simulink model "RC_DOB_mdl"  (Simulink 9.1)
settings: Solver=ode3  StartTime=0.0  StopTime=NmaxTs*Ts  FixedStep=Ts  RelTol=1e-3  EnableMultiTasking=on
values from neighbouring files (symbols this model uses):
  alpha_end = 0.999    [main_RC_DOB.m]
  alpha_init = 0    [main_RC_DOB.m]
  alpha_judge = 0.01    [main_RC_DOB.m]
  alpha_middle = 0.99    [main_RC_DOB.m]
  alpha_rate1 = 0.9    [main_RC_DOB.m]
  alpha_rate2 = 0.95    [main_RC_DOB.m]
  codeQ_gain = 0    [main_RC_DOB.m]
  d_DOB = PnZPETinverse.delaySteps    [main_RC_DOB.m]
  filterQ_gain = 1    [main_RC_DOB.m]
  g_flutter = 1    [main_RC_DOB.m]
  g_nb = 1    [main_RC_DOB.m]
  g_rro = 1    [main_RC_DOB.m]
  g_sensor = 1    [main_RC_DOB.m]
  g_torque = 1    [main_RC_DOB.m]
  loopgain = 1+loopgain_pt(jj)    [main_RC_DOB.m]
  m = d_DOB    [main_RC_DOB.m]
  RRO = SetRRO(Tsim,PlantData)    [distDefine.m]
  switch_DOB = 1    [main_RC_DOB.m]
  t_NBon = NBm/120    (= 0)    [distDefine.m]
  t_Qon = (NBm+3-NBm)/120    (= 0.025)    [distDefine.m]
  Tc = Ts    [distDefine.m]
  Ts = PlantData.Ts    [distDefine.m]    (also in main_RC_DOB.m)
undefined symbols (not defined in the file or in its folder): FlutterDist, ForceDist, MNDist, n_lplp, PlantData, SensorNoise
libraries: cstblocks x6
settings Model: Creator=Max  LastModifiedBy=daw15004
settings DataIOCC: LimitDataPoints=on  SignalLoggingSaveFormat=ModelDataLogs  SignalLoggingName=sigsOut
settings OptimizationCC: ExpressionDepthLimit=2147483647  InitFltsAndDblsToZero=on
settings DebuggingCC: SaveWithParameterizedLinksMsg=none  SignalResolutionControl=TryResolveAllWithWarning  MultiTaskDSMMsg=warning  MultiTaskCondExecSysMsg=none  FcnCallInpInsideContextMsg=warning  StateNameClashWarn=warning
settings HardwareCC: TargetUnknown=on
settings SFSimCC: SimParseCustomCode=off
settings GRTTargetCC: GeneratePreprocessorConditionals=Disable all
settings ConfigComp: CovSFcnEnable=off

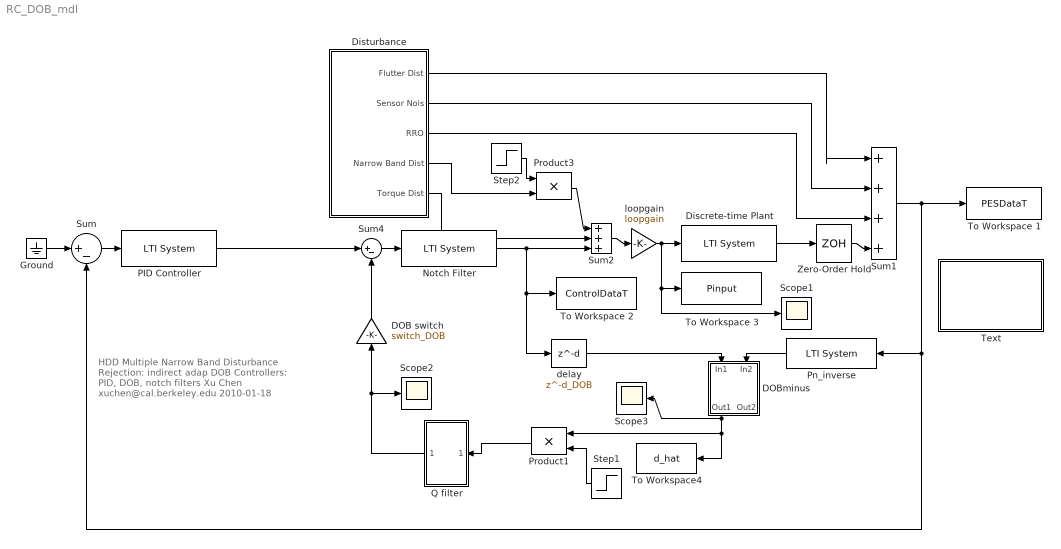
== system RC_DOB_mdl ==
  note: HDD Multiple Narrow Band
      | Disturbance Rejection: indirect adap DOB
      | Controllers: PID, DOB, notch filters
      | Xu Chen xuchen@cal.berkeley.edu
      | 2010-01-18
  DOB switch : Gain  Gain=switch_DOB  SaturateOnIntegerOverflow=on  OutDataTypeStr=Inherit: Same as input  ParamDataTypeStr=Inherit: Same as input
  DOBminus : Subsystem
  Discrete-time Plant : cstblocks/LTI System  sys=sysd_P  IC=0
  Disturbance : Subsystem
  Ground : Ground
  Notch Filter : cstblocks/LTI System  sys=sys_C2  IC=[]
  PID Controller : cstblocks/LTI System  sys=sys_C1  IC=[]
  Pn_inverse : cstblocks/LTI System  sys=G_n_inv0  IC=[]
  Product1 : Product  SaturateOnIntegerOverflow=on  OutDataTypeStr=Inherit: Same as first input
  Product3 : Product  SaturateOnIntegerOverflow=on  OutDataTypeStr=Inherit: Same as first input
  Q filter : Subsystem
  Scope1 : Scope
  Scope2 : Scope
  Scope3 : Scope
  Step1 : Step  Time=t_Qon  SampleTime=Ts
  Step2 : Step  Time=t_NBon  SampleTime=Ts
  Sum : Sum  Inputs=|+-  SaturateOnIntegerOverflow=on
  Sum1 : Sum  Inputs=+++|+  SaturateOnIntegerOverflow=on
  Sum2 : Sum  Inputs=+++  SaturateOnIntegerOverflow=on
  Sum4 : Sum  Inputs=|+-
  Text : Subsystem
      mask Display: disp('Double click here\n for help to run\nthis simulation')
  To Workspace 1 : ToWorkspace  VariableName=PESDataT  SaveFormat=Structure With Time  SampleTime=Ts
      settings: MaxDataPoints=NmaxTs
  To Workspace 2 : ToWorkspace  VariableName=ControlDataT  SaveFormat=Structure With Time  SampleTime=Tc
      settings: MaxDataPoints=NmaxTc
  To Workspace 3 : ToWorkspace  VariableName=Pinput  SaveFormat=Structure With Time  SampleTime=Tc
      settings: MaxDataPoints=NmaxTc
  To Workspace4 : ToWorkspace  VariableName=d_hat  SaveFormat=Structure With Time  SampleTime=-1
  Zero-Order Hold : ZeroOrderHold  SampleTime=Ts
  delay : Delay  DelayLength=d_DOB  InputProcessing=Inherited
  loopgain : Gain  Gain=loopgain  SaturateOnIntegerOverflow=on  OutDataTypeStr=Inherit: Same as input  ParamDataTypeStr=Inherit: Same as input
  wires:
  Ground/1 -> Sum/1
  Sum/1 -> PID Controller/1
  Sum1/1 -> To Workspace 1/1, Pn_inverse/1, Sum/2
  Disturbance/2(Sensor Nois) -> Sum1/2
  Disturbance/1(Flutter Dist) -> Sum1/1
  Disturbance/3(RRO) -> Sum1/3
  loopgain/1 -> Discrete-time Plant/1, To Workspace 3/1, Scope1/1
  Discrete-time Plant/1 -> Zero-Order Hold/1
  Zero-Order Hold/1 -> Sum1/4
  PID Controller/1 -> Sum4/1
  DOB switch/1 -> Sum4/2
  Sum2/1 -> loopgain/1
  Step2/1 -> Product3/1
  Disturbance/4(Narrow Band Dist) -> Product3/2
  Product3/1 -> Sum2/1
  Disturbance/5(Torque Dist) -> Sum2/2
  Sum4/1 -> Notch Filter/1
  Step1/1 -> Product1/2
  Product1/1 -> Q filter/1(In1)
  Q filter/1(Out1) -> DOB switch/1, Scope2/1
  delay/1 -> DOBminus/1(In1)
  Pn_inverse/1 -> DOBminus/2(In2)
  DOBminus/1(Out1) -> Scope3/1, Product1/1, To Workspace4/1
  Notch Filter/1 -> Sum2/3, To Workspace 2/1, delay/1

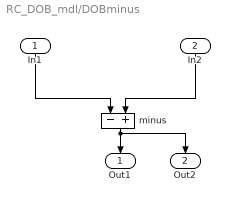
== system RC_DOB_mdl/DOBminus ==
  In1 : Inport
  In2 : Inport  Port=2
  minus : Sum  Inputs=-+
  Out1 : Outport
  Out2 : Outport  Port=2
  wires:
  In1/1 -> minus/1
  In2/1 -> minus/2
  minus/1 -> Out1/1, Out2/1

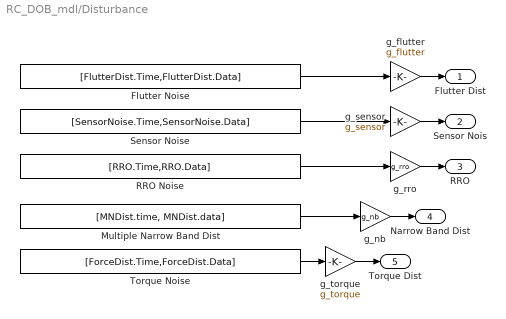
== system RC_DOB_mdl/Disturbance ==
  Flutter Noise : FromWorkspace  VariableName=[FlutterDist.Time,FlutterDist.Data]  SampleTime=FlutterDist.Ts  Interpolate=off  OutputAfterFinalValue=Setting to zero
  Multiple Narrow Band Dist : FromWorkspace  VariableName=[MNDist.time, MNDist.data]  SampleTime=MNDist.Ts  Interpolate=off  OutputAfterFinalValue=Setting to zero
  RRO Noise : FromWorkspace  VariableName=[RRO.Time,RRO.Data]  SampleTime=RRO.Ts  Interpolate=off  OutputAfterFinalValue=Setting to zero
  Sensor Noise : FromWorkspace  VariableName=[SensorNoise.Time,SensorNoise.Data]  SampleTime=SensorNoise.Ts  Interpolate=off  OutputAfterFinalValue=Setting to zero
  Torque Noise : FromWorkspace  VariableName=[ForceDist.Time,ForceDist.Data]  SampleTime=ForceDist.Ts  Interpolate=off  OutputAfterFinalValue=Setting to zero
  g_flutter : Gain  Gain=g_flutter  SaturateOnIntegerOverflow=on  OutDataTypeStr=Inherit: Same as input  ParamDataTypeStr=Inherit: Same as input
  g_nb : Gain  Gain=g_nb  SaturateOnIntegerOverflow=on  OutDataTypeStr=Inherit: Same as input  ParamDataTypeStr=Inherit: Same as input
  g_rro : Gain  Gain=g_rro  SaturateOnIntegerOverflow=on  OutDataTypeStr=Inherit: Same as input  ParamDataTypeStr=Inherit: Same as input
  g_sensor : Gain  Gain=g_sensor  SaturateOnIntegerOverflow=on  OutDataTypeStr=Inherit: Same as input  ParamDataTypeStr=Inherit: Same as input
  g_torque : Gain  Gain=g_torque  SaturateOnIntegerOverflow=on  OutDataTypeStr=Inherit: Same as input  ParamDataTypeStr=Inherit: Same as input
  Flutter Dist : Outport
  Sensor Nois : Outport  Port=2
  RRO : Outport  Port=3
  Narrow Band Dist : Outport  Port=4
  Torque Dist : Outport  Port=5
  wires:
  Multiple Narrow Band Dist/1 -> g_nb/1
  RRO Noise/1 -> g_rro/1
  Flutter Noise/1 -> g_flutter/1
  Sensor Noise/1 -> g_sensor/1
  Torque Noise/1 -> g_torque/1
  g_flutter/1 -> Flutter Dist/1
  g_sensor/1 -> Sensor Nois/1
  g_rro/1 -> RRO/1
  g_nb/1 -> Narrow Band Dist/1
  g_torque/1 -> Torque Dist/1

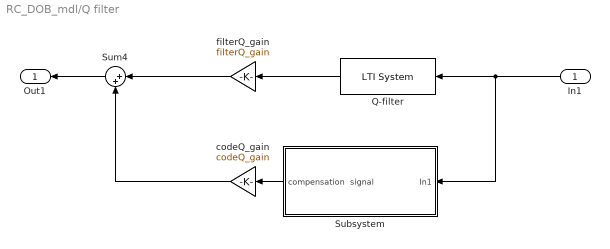
== system RC_DOB_mdl/Q filter ==
  In1 : Inport
  Q-filter : cstblocks/LTI System  sys=Q  IC=[]
  Subsystem : Subsystem
  Sum4 : Sum  Inputs=|++
  codeQ_gain : Gain  Gain=codeQ_gain  SaturateOnIntegerOverflow=on  OutDataTypeStr=Inherit: Same as input  ParamDataTypeStr=Inherit: Same as input
  filterQ_gain : Gain  Gain=filterQ_gain  SaturateOnIntegerOverflow=on  OutDataTypeStr=Inherit: Same as input  ParamDataTypeStr=Inherit: Same as input
  Out1 : Outport
  wires:
  In1/1 -> Q-filter/1, Subsystem/1(In1)
  Q-filter/1 -> filterQ_gain/1
  Subsystem/1(compensation  signal) -> codeQ_gain/1
  filterQ_gain/1 -> Sum4/1
  Sum4/1 -> Out1/1
  codeQ_gain/1 -> Sum4/2

== system RC_DOB_mdl/Text ==
  note: 3). The initial estimates (the initial conditions for the
      | integrator in the estimation algorithm block)
  note: 2). The adaptive gains (the parameters Gain and Gain1
      | in the estimation algorithm block)
  note: You can change the following parameters before
      | running the simulation and see their effects on the
      | estimator performance:
  note: This simulink program is used to implement the adaptive parallel
      | estimator in Multiple narrow band disturbance rejection.

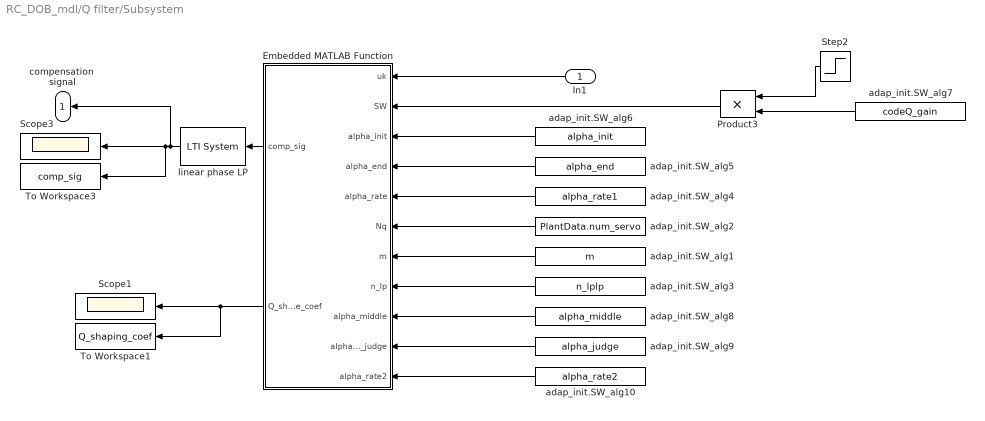
== system RC_DOB_mdl/Q filter/Subsystem ==
  In1 : Inport
  Embedded MATLAB Function : MATLAB Function  TreatAsAtomicUnit=on
  Product3 : Product  SaturateOnIntegerOverflow=on  OutDataTypeStr=Inherit: Same as first input
  Scope1 : Scope
  Scope3 : Scope
  Step2 : Step  Time=t_Qon  SampleTime=Ts
  To Workspace1 : ToWorkspace  VariableName=Q_shaping_coef  SaveFormat=Structure With Time  SampleTime=-1
  To Workspace3 : ToWorkspace  VariableName=comp_sig  SaveFormat=Structure With Time  SampleTime=-1
  adap_init.SW_alg1 : Constant  Value=m
  adap_init.SW_alg10 : Constant  Value=alpha_rate2
  adap_init.SW_alg2 : Constant  Value=PlantData.num_servo
  adap_init.SW_alg3 : Constant  Value=n_lplp
  adap_init.SW_alg4 : Constant  Value=alpha_rate1
  adap_init.SW_alg5 : Constant  Value=alpha_end
  adap_init.SW_alg6 : Constant  Value=alpha_init
  adap_init.SW_alg7 : Constant  Value=codeQ_gain
  adap_init.SW_alg8 : Constant  Value=alpha_middle
  adap_init.SW_alg9 : Constant  Value=alpha_judge
  linear phase LP : cstblocks/LTI System  sys=LPLP  IC=[]
  compensation  signal : Outport
  wires:
  Embedded MATLAB Function/1(comp_sig) -> linear phase LP/1
  Embedded MATLAB Function/2(Q_shape_coef) -> To Workspace1/1, Scope1/1
  In1/1 -> Embedded MATLAB Function/1(uk)
  adap_init.SW_alg6/1 -> Embedded MATLAB Function/3(alpha_init)
  adap_init.SW_alg5/1 -> Embedded MATLAB Function/4(alpha_end)
  adap_init.SW_alg4/1 -> Embedded MATLAB Function/5(alpha_rate)
  adap_init.SW_alg2/1 -> Embedded MATLAB Function/6(Nq)
  adap_init.SW_alg1/1 -> Embedded MATLAB Function/7(m)
  adap_init.SW_alg3/1 -> Embedded MATLAB Function/8(n_lp)
  linear phase LP/1 -> compensation  signal/1, Scope3/1, To Workspace3/1
  Step2/1 -> Product3/1
  adap_init.SW_alg7/1 -> Product3/2
  Product3/1 -> Embedded MATLAB Function/2(SW)
  adap_init.SW_alg8/1 -> Embedded MATLAB Function/9(alpha_middle)
  adap_init.SW_alg9/1 -> Embedded MATLAB Function/10(alpha_convg_judge)
  adap_init.SW_alg10/1 -> Embedded MATLAB Function/11(alpha_rate2)

== matlab function Q filter/Subsystem/Embedded MATLAB Function ==
  data: uk input double; comp_sig output double; SW input double; Q_shape_coef output double; alpha_init input double; alpha_end input double; alpha_rate input double; Nq input double; m input double; n_lp input double; alpha_middle input double; alpha_convg_judge input double; alpha_rate2 input double
function [...
    comp_sig    ,...
    Q_shape_coef]...
    = Q(...
    uk,...
    SW,...
    alpha_init,     alpha_end,      alpha_rate,...
    Nq, m, n_lp, alpha_middle, alpha_convg_judge, alpha_rate2...
    ) %#eml
persistent N ...
    x       y           ...
    alpha   iter        SW_TUNE     flag_alpha_stage1...
    %
% Code implementation of Q in RC_DOB, with dynamic shaping coefficients
%
% Xu Chen maxchen@berkeley.edu
% initial version: 2011-10-16
%
% SW_TUNE:
%           if on, the code includes an addditional shaping coeff beta
%           in the Q filter adaptation
%

if isempty(N)
    if 1
        N = 220;
    else
        N = Nq;
    end
    
    SW_TUNE                 = 0;
    
    %     N_vec   = uint16(2*N);
    %     x       = zeros(N_vec,1);
    %     x_ori   = zeros(N_vec,1);
    %     c       = zeros(N_vec,1);
    x       = (zeros(N,1));
    y       = 0;
    
    alpha       = alpha_init;
    comp_sig = 0;
    iter    = 0;
    flag_alpha_stage1 = 1;
end
if SW == 0
    %========= Adaptation turned off. ==========
    % update observation vector
    if 1 % 2011-10-16 make it comparable to filterQ
    else
    x(2:N)      = x(1:N-1);
    x(1)        = uk;
    end
    
    comp_sig    = 0;
else % if SW == 1
    
    if 1
        xk = uk+alpha^N*(x(N)-uk);
    else
        xk = (1-alpha^N)*uk+alpha^N*x(N);
    end
    y = x(N-m-n_lp);
    
    if alpha_middle == alpha_end
        alpha = alpha_end - (alpha_end-alpha) * alpha_rate; 
    else
        if flag_alpha_stage1
            delta_alpha = alpha_middle - (alpha_middle-alpha) * alpha_rate - alpha;
            % delta_alpha should be less than zero since alpha_init > alpha_middle by design
            if delta_alpha/(alpha_init-alpha_middle) > - alpha_convg_judge%0.001
                flag_alpha_stage1 = 0;
            end
            alpha = alpha + delta_alpha;
        else% alpha stage two
            alpha = alpha_end - (alpha_end-alpha) * alpha_rate2; % use a slower alpha_rate2
        end
    end
    iter = iter + 1; % iteration update
    
    % =======output========
    x(2:N) = x(1:N-1);
    x(1) = xk;
    % some gain scheduling if necessary
    if SW_TUNE
        if y > 10
            y = 10;
        end
    else
        
    end
    comp_sig = y;
end
Q_shape_coef            = alpha;
